simulink model "sgf_turtlebot_swarm"  (R2026a)
settings: Solver=ode4  StopTime=90  FixedStep=0.004
settings Model: Creator=Kshitiz  LastModifiedBy=Kshitiz

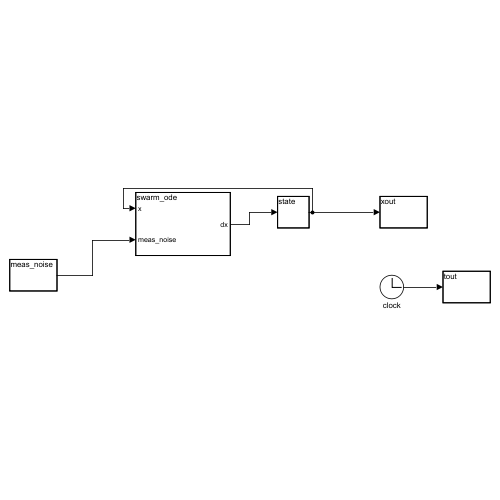
[thumbnail: Simulink's stored preview of the top-level diagram]
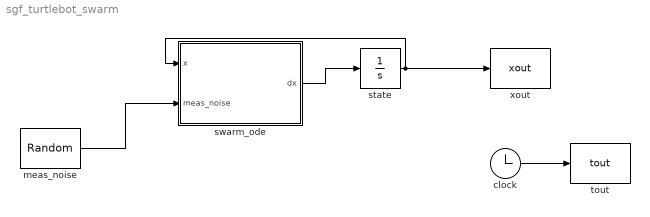
== system sgf_turtlebot_swarm ==
  clock : Clock
  meas_noise : RandomNumber  Mean=[0;0;0;0;0;0;0;0]  Variance=[0;0;0;0;0;0;0;0]  Seed=[1;2;3;4;5;6;7;8]  SampleTime=0.004
  state : Integrator  InitialCondition=[10.5;9.9194;5.5;-0.6872;-4.5;-4.3995;5.5;17.5208;5.5;9.9194;13;11.6872;5.5;-4.3995;-10;-6.5208;0;0;0;0;0;0;0;0]
  swarm_ode : MATLAB Function  TreatAsAtomicUnit=on
  tout : ToWorkspace  VariableName=tout  SampleTime=-1
  xout : ToWorkspace  VariableName=xout  SampleTime=-1
  wires:
  swarm_ode/1(dx) -> state/1
  state/1 -> swarm_ode/1(x), xout/1
  meas_noise/1 -> swarm_ode/2(meas_noise)
  clock/1 -> tout/1

== matlab function sgf_turtlebot_swarm/swarm_ode ==
  data: x input; dx output; meas_noise input
function dx = swarm_ode(x, meas_noise)
%#codegen
% Auto-generated by build_turtlebot_simulink_model. Do not edit by hand.
% meas_noise: n-vector of additive measurement noise (0 when noise-free).
n = 8;
r = 2;
R = 2;
kappa = 1;
Dmax = 12;
alpha = 10;
beta = 0.05;
noise_bound = 0.2;
eps_bl = 0.2;
src = [5.5 5.5];
adj = [0 1 0 0 0 0 0 1;1 0 1 0 0 0 0 0;0 1 0 1 0 0 0 0;0 0 1 0 1 0 0 0;0 0 0 1 0 1 0 0;0 0 0 0 1 0 1 0;0 0 0 0 0 1 0 1;1 0 0 0 0 0 1 0];
phi = [1 0;0.707106781186548 0.707106781186547;6.12323399573677e-17 1;-0.707106781186547 0.707106781186548;-1 1.22464679914735e-16;-0.707106781186548 -0.707106781186547;-1.83697019872103e-16 -1;0.707106781186547 -0.707106781186548];
px = x(1:n);
py = x(n+1:2*n);
th = x(2*n+1:3*n);
sx = px + r .* cos(th);
sy = py + r .* sin(th);
zx = sx - R .* phi(:,1);
zy = sy - R .* phi(:,2);
dx = zeros(3*n, 1);
for i = 1:n
    fx = 0.0;
    fy = 0.0;
    for j = 1:n
        if adj(i,j) ~= 0
            fx = fx + alpha * ssign(zx(j) - zx(i), eps_bl);
            fy = fy + alpha * ssign(zy(j) - zy(i), eps_bl);
        end
    end
    dsx = sx(i) - src(1);
    dsy = sy(i) - src(2);
    dist = sqrt(dsx*dsx + dsy*dsy);
    if dist < Dmax
        sigma = kappa * (dsx*dsx + dsy*dsy) + meas_noise(i);
    else
        sigma = kappa * Dmax * Dmax + noise_bound;
    end
    fx = fx - (2*beta/R) * sigma * phi(i,1);
    fy = fy - (2*beta/R) * sigma * phi(i,2);
    c = cos(th(i));
    s = sin(th(i));
    v = c*fx + s*fy;
    om = (-s*fx + c*fy) / r;
    dx(i)       = v * c;
    dx(n+i)     = v * s;
    dx(2*n+i)   = om;
end
end

function y = ssign(d, eps)
% Component-wise signum, or boundary-layer saturation sat(d/eps) when eps > 0.
if eps > 0
    y = max(min(d / eps, 1.0), -1.0);
else
    y = sign(d);
end
end
